simulink subsystem "matrixCoFactors"  (R2024b)
settings: Solver=VariableStepAuto  StartTime=0.0  StopTime=10.0  RelTol=1e-3
settings Model: Creator=ricca  LastModifiedBy=ricca

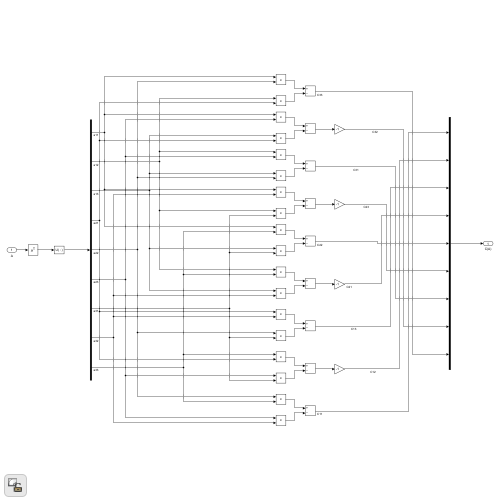
[thumbnail: Simulink's stored preview of the top-level diagram]
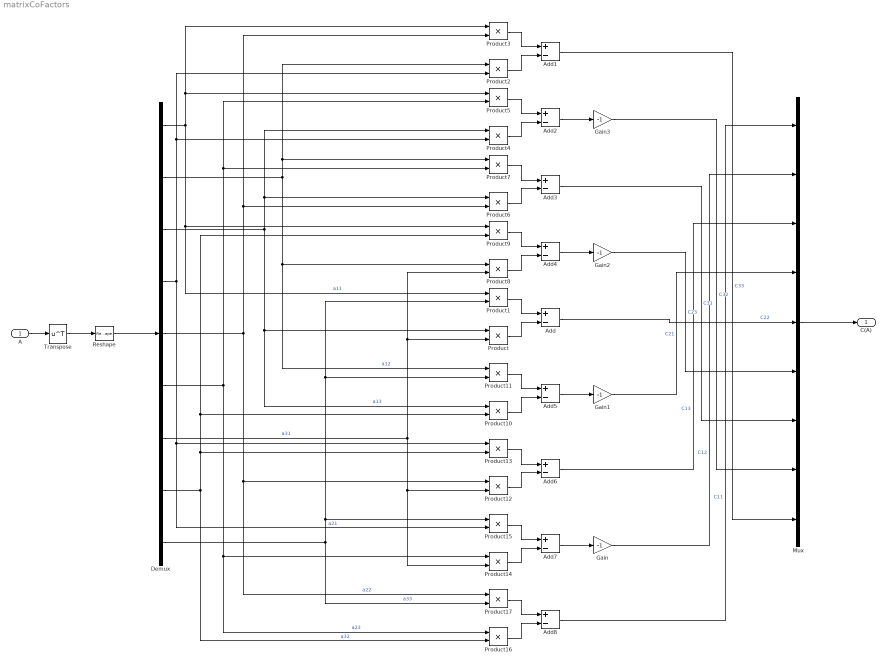
== system matrixCoFactors ==
  A : Inport
  Add{,1..8} (9 alike) : Sum  Inputs=+-
  Demux : Demux  Outputs=9
  Gain{,1..3} (4 alike) : Gain  Gain=-1
  Mux : Mux  Inputs=9
  Product{,1..17} (18 alike) : Product
  Reshape : Reshape
  Transpose : Math  Operator=transpose
  C(A) : Outport
  wires:
  A/1 -> Transpose/1
  Demux/1 -> Product1/1, Product9/1, Product5/1, Product3/1  "a11"
  Demux/2 -> Product11/1, Product8/1, Product7/1, Product2/1  "a12"
  Demux/3 -> Product/1, Product10/1, Product6/1, Product4/1  "a13"
  Demux/4 -> Product15/2, Product13/1, Product4/2, Product2/2  "a21"
  Demux/5 -> Product17/1, Product12/1, Product6/2, Product3/2  "a22"
  Demux/6 -> Product14/1, Product16/1, Product7/2, Product5/2  "a23"
  Demux/7 -> Product14/2, Product12/2, Product/2, Product8/2  "a31"
  Demux/8 -> Product16/2, Product13/2, Product10/2, Product9/2  "a32"
  Demux/9 -> Product17/2, Product15/1, Product11/2, Product1/2  "a33"
  Product1/1 -> Add/1
  Product/1 -> Add/2
  Add/1 -> Mux/5  "C22"
  Product3/1 -> Add1/1
  Add1/1 -> Mux/9  "C33"
  Product2/1 -> Add1/2
  Product5/1 -> Add2/1
  Add2/1 -> Gain3/1
  Product4/1 -> Add2/2
  Product7/1 -> Add3/1
  Add3/1 -> Mux/7  "C31"
  Product6/1 -> Add3/2
  Product9/1 -> Add4/1
  Add4/1 -> Gain2/1
  Product8/1 -> Add4/2
  Product11/1 -> Add5/1
  Add5/1 -> Gain1/1
  Product10/1 -> Add5/2
  Product13/1 -> Add6/1
  Add6/1 -> Mux/3  "C13"
  Product12/1 -> Add6/2
  Product15/1 -> Add7/1
  Add7/1 -> Gain/1
  Product14/1 -> Add7/2
  Product17/1 -> Add8/1
  Add8/1 -> Mux/1  "C11"
  Product16/1 -> Add8/2
  Gain/1 -> Mux/2  "C12"
  Gain1/1 -> Mux/4  "C21"
  Gain2/1 -> Mux/6  "C23"
  Gain3/1 -> Mux/8  "C32"
  Mux/1 -> C(A)/1
  Reshape/1 -> Demux/1
  Transpose/1 -> Reshape/1
